simulink model "drone"  (Simulink 6.1)
settings: Solver=ode4  StartTime=0.0  StopTime=15  FixedStep=1e-2  RelTol=1e-3
values from neighbouring files (symbols this model uses):
  Caero = 0    [BACKUP.mat]
  Cfrot = 0.05    [BACKUP.mat]
  Cpert = 0    [BACKUP.mat]
  DZOrientation = 0.05    [BACKUP.mat]
  ExposantFacteurAngulaire = 1    [BACKUP.mat]
  Faero = 0.8    [BACKUP.mat]
  Fpert = 0    [BACKUP.mat]
  FrotorSat = 5    [BACKUP.mat]
  InertieRotor = [0.00025  0  0; 0  0.005  0; 0  0  0.005]    [BACKUP.mat]
  KdAttitude = 0.8    [BACKUP.mat]
  KddAttitude = 0.1    [BACKUP.mat]
  KddPosition = 0.01    [BACKUP.mat]
  KdOrientation = 0.08    [BACKUP.mat]
  KdPosition = 0.5    [BACKUP.mat]
  KiAttitude = 0.001    [BACKUP.mat]
  KiOrientation = 0.02    [BACKUP.mat]
  KiPosition = 0.1    [BACKUP.mat]
  KpAttitude = 20    [BACKUP.mat]
  KpOrientation = 60    [BACKUP.mat]
  KpPosition = 50    [BACKUP.mat]
  l = 0.32    [BACKUP.mat]
  TFrotor = 0.3    [BACKUP.mat]
  Tpert = 1    [BACKUP.mat]
undefined symbols (not defined in the file or in its folder): sigbuilder_block
libraries: mblibv1 x29, simulink x20, aerolibutil x3, aerolibtransform2 x2
settings Model: LastModifiedBy=Vincent
settings OptimizationCC: InlineParams=on
settings DebuggingCC: SolverPrmCheckMsg=warning
settings SimMechanicsCC: VisOnUpdateDiagram=on  VisDuringSimulation=on

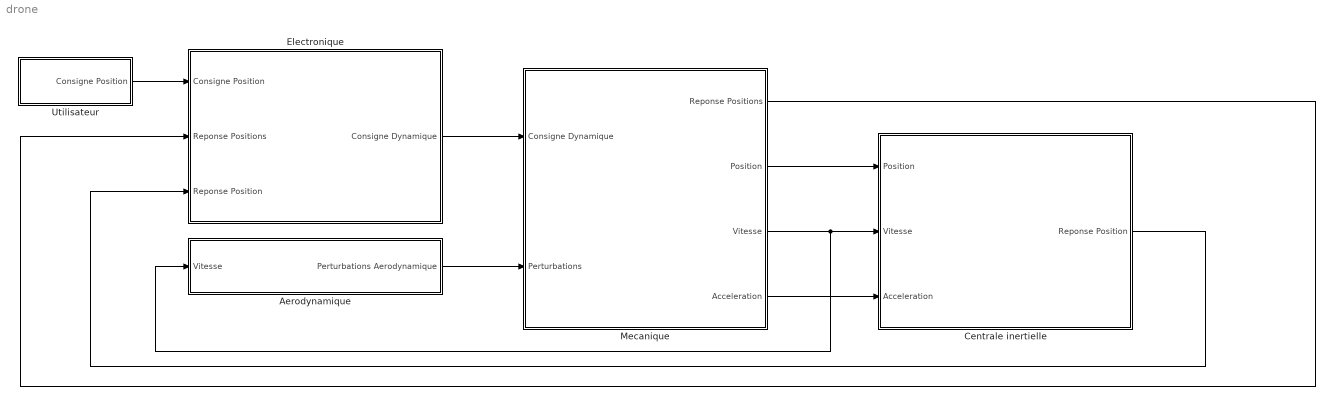
== system drone ==
  Aerodynamique : Subsystem
  Centrale inertielle : Subsystem
  Electronique : Subsystem
  Mecanique : Subsystem
  Utilisateur : Subsystem
  wires:
  Mecanique/1(Reponse Positions) -> Electronique/2(Reponse Positions)
  Electronique/1(Consigne Dynamique) -> Mecanique/1(Consigne Dynamique)
  Aerodynamique/1(Perturbations Aerodynamique) -> Mecanique/2(Perturbations)
  Utilisateur/1(Consigne Position) -> Electronique/1(Consigne Position)
  Mecanique/2(Position) -> Centrale inertielle/1(Position)
  Centrale inertielle/1(Reponse Position) -> Electronique/3(Reponse Position)
  Mecanique/4(Acceleration) -> Centrale inertielle/3(Acceleration)
  Mecanique/3(Vitesse) -> Centrale inertielle/2(Vitesse), Aerodynamique/1(Vitesse)

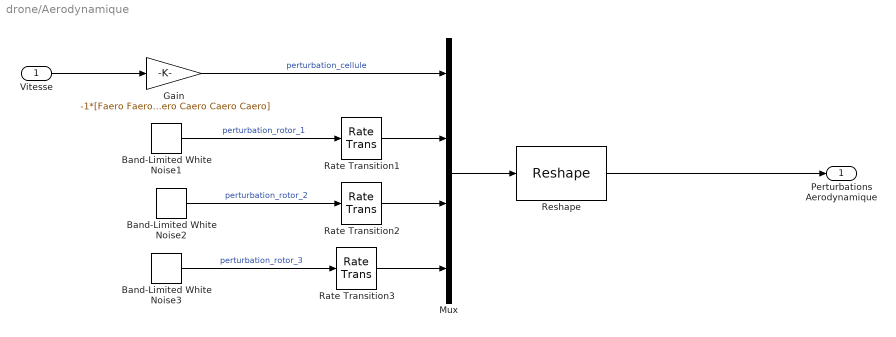
== system drone/Aerodynamique ==
  Vitesse : Inport  Port=1  LatchInput=off
  Band-Limited White Noise1 : simulink/Sources/Band-Limited White Noise  Cov=[Fpert Fpert Fpert Cpert Cpert Cpert]  Ts=Tpert  seed=rand(6,1)*1e5
  Band-Limited White Noise2 : simulink/Sources/Band-Limited White Noise  Cov=[Fpert Fpert Fpert Cpert Cpert Cpert]  Ts=Tpert  seed=rand(6,1)*1e5
  Band-Limited White Noise3 : simulink/Sources/Band-Limited White Noise  Cov=[Fpert Fpert Fpert Cpert Cpert Cpert]  Ts=Tpert  seed=rand(6,1)*1e5
  Gain : Gain  Gain=-1*[Faero Faero Faero Caero Caero Caero]
  Mux : Mux
  Rate Transition1 : RateTransition
  Rate Transition2 : RateTransition
  Rate Transition3 : RateTransition
  Reshape : simulink/Math Operations/Reshape  OutputDimensionality=1-D array  OutputDimensions=[6,4]
  Perturbations Aerodynamique : Outport
      settings: BusObject=perturbations
  wires:
  Band-Limited White Noise1/1 -> Rate Transition1/1  "perturbation_rotor_1"
  Band-Limited White Noise2/1 -> Rate Transition2/1  "perturbation_rotor_2"
  Band-Limited White Noise3/1 -> Rate Transition3/1  "perturbation_rotor_3"
  Gain/1 -> Mux/1  "perturbation_cellule"
  Mux/1 -> Reshape/1
  Reshape/1 -> Perturbations Aerodynamique/1
  Vitesse/1 -> Gain/1
  Rate Transition1/1 -> Mux/2
  Rate Transition2/1 -> Mux/3
  Rate Transition3/1 -> Mux/4

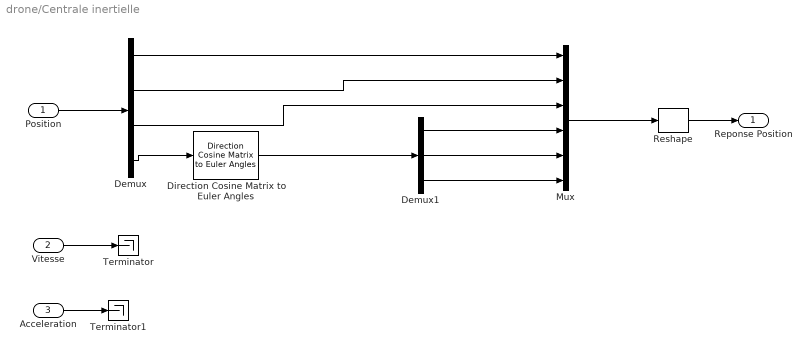
== system drone/Centrale inertielle ==
  Position : Inport  Port=1  LatchInput=off
      settings: BusObject=couples_moteurs
  Vitesse : Inport  Port=2  LatchInput=off
      settings: BusObject=couples_moteurs
  Acceleration : Inport  Port=3  LatchInput=off
      settings: BusObject=couples_moteurs
  Demux : Demux
  Demux1 : Demux  Outputs=3
  Direction Cosine Matrix to Euler Angles : aerolibtransform2/Direction Cosine Matrix to Euler Angles
  Mux : Mux  Inputs=6
  Reshape : simulink/Math Operations/Reshape  OutputDimensionality=1-D array  OutputDimensions=[1,1]
  Terminator : Terminator
  Terminator1 : Terminator
  Reponse Position : Outport
      settings: BusObject=reponse_generale
  wires:
  Position/1 -> Demux/1
  Mux/1 -> Reshape/1
  Reshape/1 -> Reponse Position/1
  Demux/4 -> Direction Cosine Matrix to Euler Angles/1
  Demux/1 -> Mux/1
  Demux/2 -> Mux/2
  Demux/3 -> Mux/3
  Demux1/1 -> Mux/4
  Demux1/2 -> Mux/5
  Demux1/3 -> Mux/6
  Direction Cosine Matrix to Euler Angles/1 -> Demux1/1
  Vitesse/1 -> Terminator/1
  Acceleration/1 -> Terminator1/1

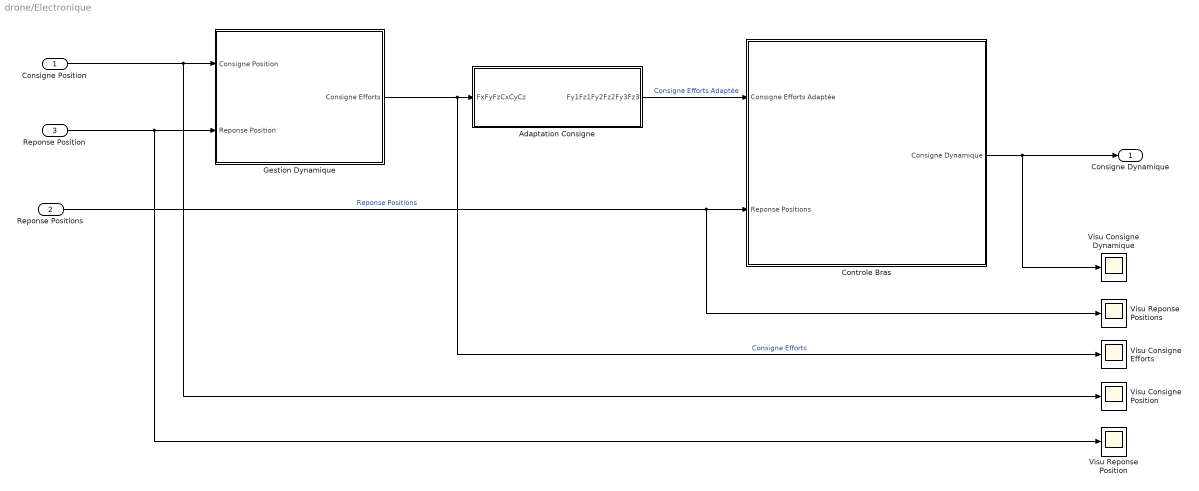
== system drone/Electronique ==
  Consigne Position : Inport  Port=1  LatchInput=off
      settings: BusObject=consigne_generale
  Reponse Positions : Inport  Port=2  LatchInput=off
      settings: BusObject=angles_moteurs
  Reponse Position : Inport  Port=3  LatchInput=off
      settings: BusObject=reponse_generale
  Adaptation Consigne : Subsystem
  Controle Bras : Subsystem
  Gestion Dynamique : Subsystem
  Visu Consigne Dynamique : Scope
      settings: YMin=-6  YMax=6  SaveName=ScopeData3
  Visu Consigne Efforts : Scope
      settings: YMin=-3.5  YMax=4.5  SaveName=ScopeData4
  Visu Consigne Position : Scope
      settings: YMin=-1  YMax=2
  Visu Reponse Position : Scope
      settings: YMin=-1.5  YMax=10
  Visu Reponse Positions : Scope
      settings: YMin=-2  YMax=3.25  SaveName=ScopeData2
  Consigne Dynamique : Outport
      settings: BusObject=couples_moteurs
  wires:
  Consigne Position/1 -> Gestion Dynamique/1(Consigne Position), Visu Consigne Position/1
  Reponse Positions/1 -> Controle Bras/2(Reponse Positions), Visu Reponse Positions/1  "Reponse Positions"
  Adaptation Consigne/1(Fy1Fz1Fy2Fz2Fy3Fz3) -> Controle Bras/1(Consigne Efforts Adaptée)  "Consigne Efforts Adaptée"
  Controle Bras/1(Consigne Dynamique) -> Consigne Dynamique/1, Visu Consigne Dynamique/1
  Gestion Dynamique/1(Consigne Efforts) -> Adaptation Consigne/1(FxFyFzCxCyCz), Visu Consigne Efforts/1  "Consigne Efforts"
  Reponse Position/1 -> Gestion Dynamique/2(Reponse Position), Visu Reponse Position/1

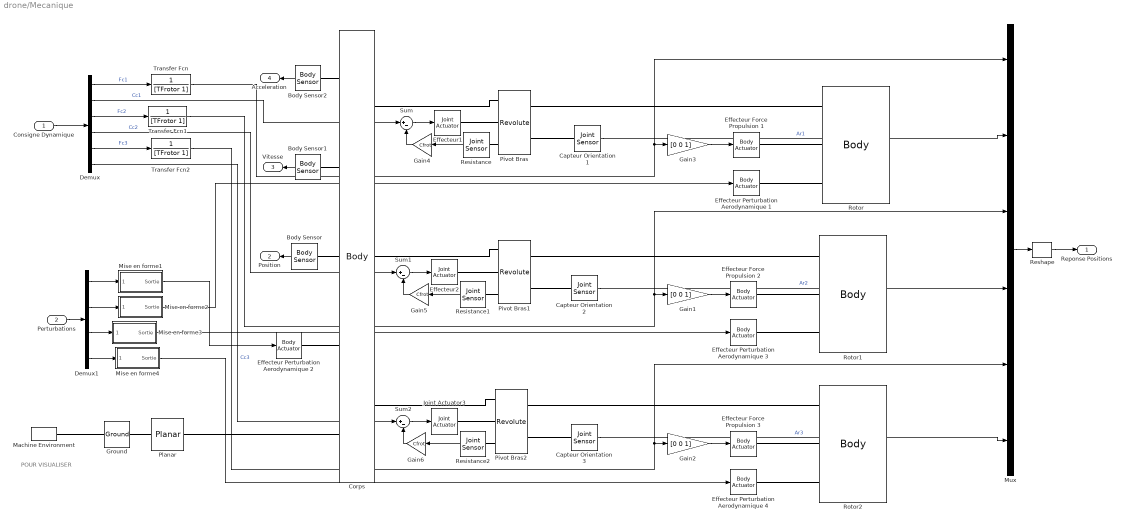
== system drone/Mecanique ==
  note: POUR VISUALISER
  Consigne Dynamique : Inport  Port=1  LatchInput=off
      settings: BusObject=couples_moteurs
  Perturbations : Inport  Port=2  LatchInput=off
      settings: BusObject=perturbations
  Body Sensor : mblibv1/Sensors &  Actuators/Body Sensor  Orientation=left  Opaque=on  PhysicalDomain=Mechanical  PortType=blob  Muxed=on  Pose=on  Angle=on  AngleUnits=deg  ArcVelocity=off  ArcVelocityUnits=deg/s  ArcAcceleration=off  ArcAccelerationUnits=deg/s^2  CoordPosition=on  CoordPositionUnits=m  Velocity=off  VelocityUnits=m/s  Acceleration=off  AccelerationUnits=m/s^2  Quaternion=on  QuaternionDT=off  QuaternionDDT=off  QuaternionUnits=off  OutputVector=[ 3 9 ]  ActiveIO=on  Width=12  DialogClass=MechanicalSensorBlock  ReferenceFrame=Absolute (World)
  Body Sensor1 : mblibv1/Sensors &  Actuators/Body Sensor  Orientation=left  Opaque=on  PhysicalDomain=Mechanical  PortType=blob  Muxed=on  Pose=off  Angle=on  AngleUnits=deg  ArcVelocity=on  ArcVelocityUnits=rad/s  ArcAcceleration=off  ArcAccelerationUnits=deg/s^2  CoordPosition=off  CoordPositionUnits=m  Velocity=on  VelocityUnits=m/s  Acceleration=off  AccelerationUnits=m/s^2  Quaternion=on  QuaternionDT=off  QuaternionDDT=off  QuaternionUnits=off  OutputVector=[ 3 3 ]  ActiveIO=on  Width=6  DialogClass=MechanicalSensorBlock  ReferenceFrame=Absolute (World)
  Body Sensor2 : mblibv1/Sensors &  Actuators/Body Sensor  Orientation=left  Opaque=on  PhysicalDomain=Mechanical  PortType=blob  Muxed=on  Pose=off  Angle=on  AngleUnits=deg  ArcVelocity=off  ArcVelocityUnits=deg/s  ArcAcceleration=on  ArcAccelerationUnits=rad/s^2  CoordPosition=off  CoordPositionUnits=m  Velocity=off  VelocityUnits=m/s  Acceleration=on  AccelerationUnits=m/s^2  Quaternion=on  QuaternionDT=off  QuaternionDDT=off  QuaternionUnits=off  OutputVector=[ 3 3 ]  ActiveIO=on  Width=6  DialogClass=MechanicalSensorBlock  ReferenceFrame=Absolute (World)
  Capteur Orientation 1 : mblibv1/Sensors &  Actuators/Joint Sensor  Opaque=on  PhysicalDomain=Mechanical  PortType=blob  Muxed=on  Pose=off  Angle=on  AngleUnits=rad  ArcVelocity=off  ArcVelocityUnits=rad/s  ArcAcceleration=off  ArcAccelerationUnits=rad/s^2  CoordPosition=on  CoordPositionUnits=m  Velocity=off  VelocityUnits=m/s  Acceleration=off  AccelerationUnits=m/s^2  Quaternion=on  QuaternionDT=off  QuaternionDDT=off  QuaternionUnits=off  OutputVector=[ 1 ]  ActiveIO=on  Width=1  DialogClass=MechanicalSensorBlock  Primitive=R1  Force=off  ForceUnits=N  Torque=off  TorqueUnits=N-m  ReferenceFrame=Absolute (INERTIAL)  ReactionSensedSide=Base  ReactionReferenceFrame=Local (Body CS)  ReactionForce=off  ReactionForceUnits=N  ReactionMoment=off  ReactionMomentUnits=N-m
  Capteur Orientation 2 : mblibv1/Sensors &  Actuators/Joint Sensor  Opaque=on  PhysicalDomain=Mechanical  PortType=blob  Muxed=on  Pose=off  Angle=on  AngleUnits=rad  ArcVelocity=off  ArcVelocityUnits=rad/s  ArcAcceleration=off  ArcAccelerationUnits=rad/s^2  CoordPosition=on  CoordPositionUnits=m  Velocity=off  VelocityUnits=m/s  Acceleration=off  AccelerationUnits=m/s^2  Quaternion=on  QuaternionDT=off  QuaternionDDT=off  QuaternionUnits=off  OutputVector=[ 1 ]  ActiveIO=on  Width=1  DialogClass=MechanicalSensorBlock  Primitive=R1  Force=off  ForceUnits=N  Torque=off  TorqueUnits=N-m  ReferenceFrame=Absolute (INERTIAL)  ReactionSensedSide=Base  ReactionReferenceFrame=Local (Body CS)  ReactionForce=off  ReactionForceUnits=N  ReactionMoment=off  ReactionMomentUnits=N-m
  Capteur Orientation 3 : mblibv1/Sensors &  Actuators/Joint Sensor  Opaque=on  PhysicalDomain=Mechanical  PortType=blob  Muxed=on  Pose=off  Angle=on  AngleUnits=rad  ArcVelocity=off  ArcVelocityUnits=rad/s  ArcAcceleration=off  ArcAccelerationUnits=rad/s^2  CoordPosition=on  CoordPositionUnits=m  Velocity=off  VelocityUnits=m/s  Acceleration=off  AccelerationUnits=m/s^2  Quaternion=on  QuaternionDT=off  QuaternionDDT=off  QuaternionUnits=off  OutputVector=[ 1 ]  ActiveIO=on  Width=1  DialogClass=MechanicalSensorBlock  Primitive=R1  Force=off  ForceUnits=N  Torque=off  TorqueUnits=N-m  ReferenceFrame=Absolute (INERTIAL)  ReactionSensedSide=Base  ReactionReferenceFrame=Local (Body CS)  ReactionForce=off  ReactionForceUnits=N  ReactionMoment=off  ReactionMomentUnits=N-m
  Corps : mblibv1/Bodies/Body  PhysicalDomain=mechanical  SubClassName=Unknown  LeftPortType=workingframe  RightPortType=workingframe  LConnTagsString=CS4|CS5|CS6|CS7|CG  RConnTagsString=CS1|CS2|CS3  DialogClass=MechanicalBodyBlock  Mass=0.2  MassUnits=kg  InertiaUnits=kg*m^2  Inertia=eye(3)  Shape=Cylinder  ShapeDims=[1 1]  ShapeUnits=m  ShapeUse=false  Density=1  DensityUnits=kg/m^3  DensityUse=false  CG=Left$CG$[0 0 0]$ADJOINING$ADJOINING$m$[0 0 0]$Euler X-Y-Z$deg$ADJOINING$true  WorkingFrames=Right$CS1$[0 0 0]$CG$CG$m$[0 0 0]$Euler Z-Y-X$deg$CG$true#Right$CS2$[0 0 0]$CG$CG$m$[120 0 0]$Euler Z-Y-X$deg$CG$true#Right$CS3$[0 0 0]$CG$CG$m$[240 0 0]$Euler Z-Y-X$deg$CG$true#Left$CS4$[0 0 0]$CG$CG$m$[0 0 0]$Euler X-Y-Z$deg$WORLD$true#Left$CS5$[0 0 0]$CG$CG$m$[0 0 0]$Euler X-Y-Z$deg$WORLD$true#Left$CS6$[0 0 0]$CG$CG$m$[0 0 0]$Euler X-Y-Z$deg$WORLD$true#Left$CS7$[0 0 0]$CG$CG$m$[0 0 0]$Euler X-Y-Z$deg$WORLD$true
  Demux : Demux  Outputs=6
  Demux1 : Demux
  Effecteur Force Propulsion 1 : mblibv1/Sensors &  Actuators/Body Actuator  Opaque=on  PhysicalDomain=Mechanical  PortType=blob  ActuationStyle=Force  AngleUnits=deg  ArcVelocityUnits=deg/s  ArcAccelerationUnits=deg/s^2  CoordPositionUnits=m  VelocityUnits=m/s  AccelerationUnits=m/s^2  ForceUnits=N  TorqueUnits=N-m  ActiveIO=on  Width=3  DialogClass=MechanicalActuatorBlock  ReferenceFrame=Local (Body CS)  Angle=off  CoordPosition=on  Force=on  Torque=off
  Effecteur Force Propulsion 2 : mblibv1/Sensors &  Actuators/Body Actuator  Opaque=on  PhysicalDomain=Mechanical  PortType=blob  ActuationStyle=Force  AngleUnits=deg  ArcVelocityUnits=deg/s  ArcAccelerationUnits=deg/s^2  CoordPositionUnits=m  VelocityUnits=m/s  AccelerationUnits=m/s^2  ForceUnits=N  TorqueUnits=N-m  ActiveIO=on  Width=3  DialogClass=MechanicalActuatorBlock  ReferenceFrame=Local (Body CS)  Angle=off  CoordPosition=on  Force=on  Torque=off
  Effecteur Force Propulsion 3 : mblibv1/Sensors &  Actuators/Body Actuator  Opaque=on  PhysicalDomain=Mechanical  PortType=blob  ActuationStyle=Force  AngleUnits=deg  ArcVelocityUnits=deg/s  ArcAccelerationUnits=deg/s^2  CoordPositionUnits=m  VelocityUnits=m/s  AccelerationUnits=m/s^2  ForceUnits=N  TorqueUnits=N-m  ActiveIO=on  Width=3  DialogClass=MechanicalActuatorBlock  ReferenceFrame=Local (Body CS)  Angle=off  CoordPosition=on  Force=on  Torque=off
  Effecteur Perturbation Aerodynamique 1 : mblibv1/Sensors &  Actuators/Body Actuator  Opaque=on  PhysicalDomain=Mechanical  PortType=blob  ActuationStyle=Force  AngleUnits=deg  ArcVelocityUnits=deg/s  ArcAccelerationUnits=deg/s^2  CoordPositionUnits=m  VelocityUnits=m/s  AccelerationUnits=m/s^2  ForceUnits=N  TorqueUnits=N-m  ActiveIO=on  Width=6  DialogClass=MechanicalActuatorBlock  ReferenceFrame=Local (Body CS)  Angle=off  CoordPosition=on  Force=on  Torque=on
  Effecteur Perturbation Aerodynamique 2 : mblibv1/Sensors &  Actuators/Body Actuator  Opaque=on  PhysicalDomain=Mechanical  PortType=blob  ActuationStyle=Force  AngleUnits=deg  ArcVelocityUnits=deg/s  ArcAccelerationUnits=deg/s^2  CoordPositionUnits=m  VelocityUnits=m/s  AccelerationUnits=m/s^2  ForceUnits=N  TorqueUnits=N-m  ActiveIO=on  Width=6  DialogClass=MechanicalActuatorBlock  ReferenceFrame=Absolute (World)  Angle=off  CoordPosition=on  Force=on  Torque=on
  Effecteur Perturbation Aerodynamique 3 : mblibv1/Sensors &  Actuators/Body Actuator  Opaque=on  PhysicalDomain=Mechanical  PortType=blob  ActuationStyle=Force  AngleUnits=deg  ArcVelocityUnits=deg/s  ArcAccelerationUnits=deg/s^2  CoordPositionUnits=m  VelocityUnits=m/s  AccelerationUnits=m/s^2  ForceUnits=N  TorqueUnits=N-m  ActiveIO=on  Width=6  DialogClass=MechanicalActuatorBlock  ReferenceFrame=Local (Body CS)  Angle=off  CoordPosition=on  Force=on  Torque=on
  Effecteur Perturbation Aerodynamique 4 : mblibv1/Sensors &  Actuators/Body Actuator  Opaque=on  PhysicalDomain=Mechanical  PortType=blob  ActuationStyle=Force  AngleUnits=deg  ArcVelocityUnits=deg/s  ArcAccelerationUnits=deg/s^2  CoordPositionUnits=m  VelocityUnits=m/s  AccelerationUnits=m/s^2  ForceUnits=N  TorqueUnits=N-m  ActiveIO=on  Width=6  DialogClass=MechanicalActuatorBlock  ReferenceFrame=Local (Body CS)  Angle=off  CoordPosition=on  Force=on  Torque=on
  Effecteur1 : mblibv1/Sensors &  Actuators/Joint Actuator  Opaque=on  PhysicalDomain=Mechanical  PortType=blob  ActuationStyle=Force  AngleUnits=deg  ArcVelocityUnits=deg/s  ArcAccelerationUnits=deg/s^2  CoordPositionUnits=m  VelocityUnits=m/s  AccelerationUnits=m/s^2  ForceUnits=N  TorqueUnits=N-m  ActiveIO=on  Width=1  DialogClass=MechanicalActuatorBlock  Primitive=R1  ReferenceFrame=Absolute (INERTIAL)
  Effecteur2 : mblibv1/Sensors &  Actuators/Joint Actuator  Opaque=on  PhysicalDomain=Mechanical  PortType=blob  ActuationStyle=Force  AngleUnits=deg  ArcVelocityUnits=deg/s  ArcAccelerationUnits=deg/s^2  CoordPositionUnits=m  VelocityUnits=m/s  AccelerationUnits=m/s^2  ForceUnits=N  TorqueUnits=N-m  ActiveIO=on  Width=1  DialogClass=MechanicalActuatorBlock  Primitive=R1  ReferenceFrame=Absolute (INERTIAL)
  Gain1 : Gain  Gain=[0 0 1]
  Gain2 : Gain  Gain=[0 0 1]
  Gain3 : Gain  Gain=[0 0 1]
  Gain4 : Gain  Orientation=left  Gain=Cfrot
  Gain5 : Gain  Orientation=left  Gain=Cfrot
  Gain6 : Gain  Orientation=left  Gain=Cfrot
  Ground : mblibv1/Bodies/Ground  Opaque=on  LeftPortType=env  RightPortType=workingframe  PhysicalDomain=Mechanical  DialogClass=GroundBlock  CoordPosition=[0 0 0]  CoordPositionUnits=m  StateVectorMgrId=-1  MachineId=[1 0]  ShowEnvPort=on
  Joint Actuator3 : mblibv1/Sensors &  Actuators/Joint Actuator  Opaque=on  PhysicalDomain=Mechanical  PortType=blob  ActuationStyle=Force  AngleUnits=deg  ArcVelocityUnits=deg/s  ArcAccelerationUnits=deg/s^2  CoordPositionUnits=m  VelocityUnits=m/s  AccelerationUnits=m/s^2  ForceUnits=N  TorqueUnits=N-m  ActiveIO=on  Width=1  DialogClass=MechanicalActuatorBlock  Primitive=R1  ReferenceFrame=Absolute (INERTIAL)
  Machine Environment : mblibv1/Bodies/Machine Environment  Tag=Factory ground  DialogController=MECH.DialogSource  Opaque=on  PortType=env  PhysicalDomain=Mechanical  DialogTemplateClass=MECH.MachineEnvironment  SyncWhenCopied=off  Gravity=[0 0 -9.81]  GravityUnits=m/s^2  GravityAsSignal=off  Dimensionality=3D Only  AnalysisType=Forward dynamics  LinearAssemblyTolerance=1e-3  LinearAssemblyToleranceUnits=m  AngularAssemblyTolerance=1e-3  AngularAssemblyToleranceUnits=rad  ConstraintSolverType=Stabilizing  ConstraintRelTolerance=1e-4  ConstraintAbsTolerance=1e-4  UseRobustSingularityHandling=off  StatePerturbationType=Fixed  PerturbationSize=1e-5  VisualizeMachine=on
  Mise en forme1 : Subsystem
  Mise en forme2 : Subsystem
  Mise en forme3 : Subsystem
  Mise en forme4 : Subsystem
  Mux : Mux  Inputs=6
  Pivot Bras : mblibv1/Joints/Revolute  PhysicalDomain=mechanical  SubClassName=Unknown  LeftPortType=blob  RightPortType=blob  LConnTagsString=__newl0|SA1|SA2  RConnTagsString=__newr0|SA1  NumSAPorts=3  CutJoint=off  MarkAsCut=off  Primitives=revolute  PrimitiveProps=R1$Base$[1 0 0]$revolute  DialogClass=JointBlock
  Pivot Bras1 : mblibv1/Joints/Revolute  PhysicalDomain=mechanical  SubClassName=Unknown  LeftPortType=blob  RightPortType=blob  LConnTagsString=__newl0|SA1|SA2  RConnTagsString=__newr0|SA1  NumSAPorts=3  CutJoint=off  MarkAsCut=off  Primitives=revolute  PrimitiveProps=R1$Base$[1 0 0]$revolute  DialogClass=JointBlock
  Pivot Bras2 : mblibv1/Joints/Revolute  PhysicalDomain=mechanical  SubClassName=Unknown  LeftPortType=blob  RightPortType=blob  LConnTagsString=__newl0|SA1|SA2  RConnTagsString=__newr0|SA1  NumSAPorts=3  CutJoint=off  MarkAsCut=off  Primitives=revolute  PrimitiveProps=R1$Base$[1 0 0]$revolute  DialogClass=JointBlock
  Planar : mblibv1/Joints/Planar  PhysicalDomain=mechanical  SubClassName=Unknown  LeftPortType=blob  RightPortType=blob  LConnTagsString=__newl0  RConnTagsString=__newr0  NumSAPorts=0  CutJoint=off  MarkAsCut=off  Primitives=prismatic_prismatic_revolute  PrimitiveProps=P1$INERTIAL$[1 0 0]$prismatic#P2$INERTIAL$[0 1 0]$prismatic#R1$INERTIAL$[0 0 1]$revolute  DialogClass=JointBlock
  Reshape : simulink/Math Operations/Reshape  OutputDimensionality=1-D array  OutputDimensions=[1,1]
  Resistance : mblibv1/Sensors &  Actuators/Joint Sensor  Orientation=left  Opaque=on  PhysicalDomain=Mechanical  PortType=blob  Muxed=on  Pose=off  Angle=off  AngleUnits=rad  ArcVelocity=on  ArcVelocityUnits=rad/s  ArcAcceleration=off  ArcAccelerationUnits=rad/s^2  CoordPosition=on  CoordPositionUnits=m  Velocity=off  VelocityUnits=m/s  Acceleration=off  AccelerationUnits=m/s^2  Quaternion=on  QuaternionDT=off  QuaternionDDT=off  QuaternionUnits=off  OutputVector=[ 1 ]  ActiveIO=on  Width=1  DialogClass=MechanicalSensorBlock  Primitive=R1  Force=off  ForceUnits=N  Torque=off  TorqueUnits=N-m  ReferenceFrame=Absolute (INERTIAL)  ReactionSensedSide=Base  ReactionReferenceFrame=Local (Body CS)  ReactionForce=off  ReactionForceUnits=N  ReactionMoment=off  ReactionMomentUnits=N-m
  Resistance1 : mblibv1/Sensors &  Actuators/Joint Sensor  Orientation=left  Opaque=on  PhysicalDomain=Mechanical  PortType=blob  Muxed=on  Pose=off  Angle=off  AngleUnits=rad  ArcVelocity=on  ArcVelocityUnits=rad/s  ArcAcceleration=off  ArcAccelerationUnits=rad/s^2  CoordPosition=on  CoordPositionUnits=m  Velocity=off  VelocityUnits=m/s  Acceleration=off  AccelerationUnits=m/s^2  Quaternion=on  QuaternionDT=off  QuaternionDDT=off  QuaternionUnits=off  OutputVector=[ 1 ]  ActiveIO=on  Width=1  DialogClass=MechanicalSensorBlock  Primitive=R1  Force=off  ForceUnits=N  Torque=off  TorqueUnits=N-m  ReferenceFrame=Absolute (INERTIAL)  ReactionSensedSide=Base  ReactionReferenceFrame=Local (Body CS)  ReactionForce=off  ReactionForceUnits=N  ReactionMoment=off  ReactionMomentUnits=N-m
  Resistance2 : mblibv1/Sensors &  Actuators/Joint Sensor  Orientation=left  Opaque=on  PhysicalDomain=Mechanical  PortType=blob  Muxed=on  Pose=off  Angle=off  AngleUnits=rad  ArcVelocity=on  ArcVelocityUnits=rad/s  ArcAcceleration=off  ArcAccelerationUnits=rad/s^2  CoordPosition=on  CoordPositionUnits=m  Velocity=off  VelocityUnits=m/s  Acceleration=off  AccelerationUnits=m/s^2  Quaternion=on  QuaternionDT=off  QuaternionDDT=off  QuaternionUnits=off  OutputVector=[ 1 ]  ActiveIO=on  Width=1  DialogClass=MechanicalSensorBlock  Primitive=R1  Force=off  ForceUnits=N  Torque=off  TorqueUnits=N-m  ReferenceFrame=Absolute (INERTIAL)  ReactionSensedSide=Base  ReactionReferenceFrame=Local (Body CS)  ReactionForce=off  ReactionForceUnits=N  ReactionMoment=off  ReactionMomentUnits=N-m
  Rotor : mblibv1/Bodies/Body  PhysicalDomain=mechanical  SubClassName=Unknown  LeftPortType=workingframe  RightPortType=workingframe  LConnTagsString=CS1|CS2|CS3  DialogClass=MechanicalBodyBlock  Mass=0.1  MassUnits=kg  InertiaUnits=kg*m^2  Inertia=InertieRotor  Shape=Cylinder  ShapeDims=[1 1]  ShapeUnits=m  ShapeUse=false  Density=1  DensityUnits=kg/m^3  DensityUse=false  CG=Left$CG$l*[1 0 0]$CS1$CS1$m$[0 0 0]$Euler X-Y-Z$deg$CS1$false  WorkingFrames=Left$CS1$[0 0 0]$ADJOINING$ADJOINING$m$[0 0 0]$Euler X-Y-Z$deg$ADJOINING$true#Left$CS2$l*[1 0 0]$CS1$CS1$m$[0 0 0]$Euler X-Y-Z$deg$CS1$true#Left$CS3$l*[1 0 0]$CS1$CS1$m$[0 0 0]$Euler X-Y-Z$deg$CS1$true
  Rotor1 : mblibv1/Bodies/Body  PhysicalDomain=mechanical  SubClassName=Unknown  LeftPortType=workingframe  RightPortType=workingframe  LConnTagsString=CS1|CS2|CS3  DialogClass=MechanicalBodyBlock  Mass=0.1  MassUnits=kg  InertiaUnits=kg*m^2  Inertia=InertieRotor  Shape=Cylinder  ShapeDims=[1 1]  ShapeUnits=m  ShapeUse=false  Density=1  DensityUnits=kg/m^3  DensityUse=false  CG=Left$CG$l*[1 0 0]$CS1$CS1$m$[0 0 0]$Euler X-Y-Z$deg$CS1$false  WorkingFrames=Left$CS1$[0 0 0]$ADJOINING$ADJOINING$m$[0 0 0]$Euler X-Y-Z$deg$ADJOINING$true#Left$CS2$l*[1 0 0]$CS1$CS1$m$[0 0 0]$Euler X-Y-Z$deg$CS1$true#Left$CS3$l*[1 0 0]$CS1$CS1$m$[0 0 0]$Euler X-Y-Z$deg$CS1$true
  Rotor2 : mblibv1/Bodies/Body  PhysicalDomain=mechanical  SubClassName=Unknown  LeftPortType=workingframe  RightPortType=workingframe  LConnTagsString=CS1|CS2|CS3  DialogClass=MechanicalBodyBlock  Mass=0.1  MassUnits=kg  InertiaUnits=kg*m^2  Inertia=InertieRotor  Shape=Cylinder  ShapeDims=[1 1]  ShapeUnits=m  ShapeUse=false  Density=1  DensityUnits=kg/m^3  DensityUse=false  CG=Left$CG$l*[1 0 0]$CS1$CS1$m$[0 0 0]$Euler X-Y-Z$deg$CS1$false  WorkingFrames=Left$CS1$[0 0 0]$ADJOINING$ADJOINING$m$[0 0 0]$Euler X-Y-Z$deg$ADJOINING$true#Left$CS2$l*[1 0 0]$CS1$CS1$m$[0 0 0]$Euler X-Y-Z$deg$CS1$true#Left$CS3$l*[1 0 0]$CS1$CS1$m$[0 0 0]$Euler X-Y-Z$deg$CS1$true
  Sum : Sum  Inputs=|+-
  Sum1 : Sum  Inputs=|+-
  Sum2 : Sum  Inputs=|+-
  Transfer Fcn : TransferFcn  Denominator=[TFrotor 1]
  Transfer Fcn1 : TransferFcn  Denominator=[TFrotor 1]
  Transfer Fcn2 : TransferFcn  Denominator=[TFrotor 1]
  Reponse Positions : Outport
      settings: BusObject=angles_moteurs
  Position : Outport  Orientation=left  Port=2
      settings: BusObject=angles_moteurs
  Vitesse : Outport  Orientation=left  Port=3
      settings: BusObject=angles_moteurs
  Acceleration : Outport  Orientation=left  Port=4
      settings: BusObject=angles_moteurs
  wires:
  Consigne Dynamique/1 -> Demux/1
  Demux/2 -> Sum/1  "Cc1"
  Demux/1 -> Transfer Fcn/1  "Fc1"
  Demux/4 -> Sum1/1  "Cc2"
  Demux/3 -> Transfer Fcn1/1  "Fc2"
  Demux/5 -> Transfer Fcn2/1  "Fc3"
  Demux/6 -> Sum2/1  "Cc3"
  Reshape/1 -> Reponse Positions/1
  Capteur Orientation 3/1 -> Mux/6  "Ar3"
  Capteur Orientation 2/1 -> Mux/4  "Ar2"
  Capteur Orientation 1/1 -> Mux/2  "Ar1"
  Mux/1 -> Reshape/1
  Gain2/1 -> Effecteur Force Propulsion 3/1
  Gain1/1 -> Effecteur Force Propulsion 2/1
  Gain3/1 -> Effecteur Force Propulsion 1/1
  Perturbations/1 -> Demux1/1
  Demux1/2 -> Mise en forme2/1(Entree)
  Demux1/3 -> Mise en forme3/1(Entree)
  Demux1/4 -> Mise en forme4/1(Entree)
  Demux1/1 -> Mise en forme1/1(Entree)
  Sum/1 -> Effecteur1/1
  Resistance/1 -> Gain4/1
  Gain4/1 -> Sum/2
  Gain5/1 -> Sum1/2
  Resistance1/1 -> Gain5/1
  Sum1/1 -> Effecteur2/1
  Gain6/1 -> Sum2/2
  Resistance2/1 -> Gain6/1
  Sum2/1 -> Joint Actuator3/1
  Transfer Fcn/1 -> Mux/1, Gain3/1
  Transfer Fcn1/1 -> Mux/3, Gain1/1
  Transfer Fcn2/1 -> Mux/5, Gain2/1
  Body Sensor/1 -> Position/1
  Body Sensor1/1 -> Vitesse/1
  Body Sensor2/1 -> Acceleration/1
  Mise en forme1/1(Sortie) -> Effecteur Perturbation Aerodynamique 2/1
  Mise en forme2/1(Sortie) -> Effecteur Perturbation Aerodynamique 1/1
  Mise en forme3/1(Sortie) -> Effecteur Perturbation Aerodynamique 3/1
  Mise en forme4/1(Sortie) -> Effecteur Perturbation Aerodynamique 4/1
  connections:
  Corps/RConn1 -- Pivot Bras/LConn1
  Pivot Bras/RConn1 -- Rotor/LConn1
  Effecteur Force Propulsion 1/RConn1 -- Rotor/LConn2
  Effecteur Perturbation Aerodynamique 1/RConn1 -- Rotor/LConn3
  Pivot Bras/RConn2 -- Capteur Orientation 1/LConn1
  Ground/RConn1 -- Planar/LConn1
  Planar/RConn1 -- Corps/LConn5
  Machine Environment/RConn1 -- Ground/LConn1
  Effecteur1/RConn1 -- Pivot Bras/LConn2
  Pivot Bras1/RConn1 -- Rotor1/LConn1
  Effecteur Force Propulsion 2/RConn1 -- Rotor1/LConn2
  Effecteur Perturbation Aerodynamique 3/RConn1 -- Rotor1/LConn3
  Pivot Bras1/RConn2 -- Capteur Orientation 2/LConn1
  Effecteur2/RConn1 -- Pivot Bras1/LConn2
  Pivot Bras2/RConn1 -- Rotor2/LConn1
  Effecteur Force Propulsion 3/RConn1 -- Rotor2/LConn2
  Effecteur Perturbation Aerodynamique 4/RConn1 -- Rotor2/LConn3
  Pivot Bras2/RConn2 -- Capteur Orientation 3/LConn1
  Joint Actuator3/RConn1 -- Pivot Bras2/LConn2
  Corps/RConn2 -- Pivot Bras1/LConn1
  Corps/RConn3 -- Pivot Bras2/LConn1
  Pivot Bras/LConn3 -- Resistance/LConn1
  Pivot Bras1/LConn3 -- Resistance1/LConn1
  Pivot Bras2/LConn3 -- Resistance2/LConn1
  Effecteur Perturbation Aerodynamique 2/RConn1 -- Corps/LConn4
  Corps/LConn3 -- Body Sensor/LConn1
  Body Sensor1/LConn1 -- Corps/LConn2
  Body Sensor2/LConn1 -- Corps/LConn1

== system drone/Utilisateur ==
  Generateur F : Subsystem  Tag=STV Subsys  LoadFcn=sigbuilder_block('load',[0 42 1080 574.5 ]);  StartFcn=sigbuilder_block('start');  StopFcn=sigbuilder_block('stop');  ClipboardFcn=sigbuilder_block('clipboard');  mask(Sigbuilder block){}
      mask help: Sigbuilder GUI
      mask init:
      | if ~strcmp(get_param(bdroot(gcbh),'SimulationStatus'),'stopped') tuvar = sigbuilder_block('maskInit'); end
      settings: CopyFcn=sigbuilder_block('copy');  DeleteFcn=sigbuilder_block('delete');  ModelCloseFcn=sigbuilder_block('modelClose');  PreSaveFcn=sigbuilder_block('preSave');  NameChangeFcn=sigbuilder_block('namechange');  OpenFcn=sigbuilder_block('open',[0 42 1080 574.5 ]);  CloseFcn=sigbuilder_block('close');
      mask Display: plot(0,0,100,100,[10,10,40,40,10],[80,20,20,80,80],[40,10],[50,50], [40,27,10],[65,72,56],[40,25,25,10],[28,28,43,43]);
  Mux : Mux  Inputs=6
  Reshape2 : simulink/Math Operations/Reshape  OutputDimensionality=1-D array  OutputDimensions=[1,1]
  Consigne Position : Outport
      settings: BusObject=consigne_generale
  wires:
  Mux/1 -> Reshape2/1
  Reshape2/1 -> Consigne Position/1
  Generateur F/1(X) -> Mux/1
  Generateur F/2(Y) -> Mux/2
  Generateur F/3(Z) -> Mux/3
  Generateur F/4(Phi) -> Mux/4
  Generateur F/5(Theta) -> Mux/5
  Generateur F/6(Psi) -> Mux/6

== system drone/Electronique/Adaptation Consigne ==
  FxFyFzCxCyCz : Inport  Port=1  LatchInput=off
  Matrice Correction : Constant  Value=[-1 -1 1 1/l 1/l 1/l]
  Matrice Transformation : Constant  Value=(1/3)*[0 2 0 0 0 1; 0 0 1 0 2 0; -sqrt(3) -1 0 0 0 1; 0 0 1 -sqrt(3) -1 0; sqrt(3) -1 0 0 0 1; 0 0 1 sqrt(3) -1 0]  VectorParams1D=off
  Product : Product  Multiplication=Matrix(*)  RndMeth=Zero
  Product1 : Product  RndMeth=Zero
  Fy1Fz1Fy2Fz2Fy3Fz3 : Outport
  wires:
  Product/1 -> Fy1Fz1Fy2Fz2Fy3Fz3/1
  Matrice Transformation/1 -> Product/1
  Matrice Correction/1 -> Product1/2
  FxFyFzCxCyCz/1 -> Product1/1
  Product1/1 -> Product/2

== system drone/Electronique/Controle Bras ==
  Consigne Efforts Adaptée : Inport  Port=1  LatchInput=off
  Reponse Positions : Inport  Port=2  LatchInput=off
  Controle Bras1 : Subsystem
  Controle Bras2 : Subsystem
  Controle Bras3 : Subsystem
  Demux1 : Demux  Outputs=6
  Demux2 : Demux  Outputs=6
  Mux : Mux  Inputs=6
  Reshape : simulink/Math Operations/Reshape  OutputDimensionality=1-D array  OutputDimensions=[1,1]
  Consigne Dynamique : Outport
  wires:
  Demux1/1 -> Controle Bras1/3(Fr)  "Fr1"
  Demux1/2 -> Controle Bras1/4(Ar)  "Ar1"
  Demux1/3 -> Controle Bras2/3(Fr)  "Fr2"
  Demux1/4 -> Controle Bras2/4(Ar)  "Ar2"
  Demux1/5 -> Controle Bras3/3(Fr)  "Fr3"
  Demux1/6 -> Controle Bras3/4(Ar)  "Ar3"
  Demux2/3 -> Controle Bras2/1(Fyc)  "Fyc2"
  Demux2/4 -> Controle Bras2/2(Fzc)  "Fzc2"
  Demux2/5 -> Controle Bras3/1(Fyc)  "Fyc3"
  Demux2/6 -> Controle Bras3/2(Fzc)  "Fzc3"
  Demux2/1 -> Controle Bras1/1(Fyc)  "Fyc1"
  Demux2/2 -> Controle Bras1/2(Fzc)  "Fzc1"
  Reponse Positions/1 -> Demux1/1
  Consigne Efforts Adaptée/1 -> Demux2/1
  Controle Bras1/1(Fc) -> Mux/1  "Fc1"
  Controle Bras1/2(Cc) -> Mux/2  "Cc1"
  Controle Bras2/1(Fc) -> Mux/3  "Fc2"
  Controle Bras2/2(Cc) -> Mux/4  "Cc2"
  Controle Bras3/1(Fc) -> Mux/5  "Fc3"
  Controle Bras3/2(Cc) -> Mux/6  "Cc3"
  Mux/1 -> Reshape/1
  Reshape/1 -> Consigne Dynamique/1

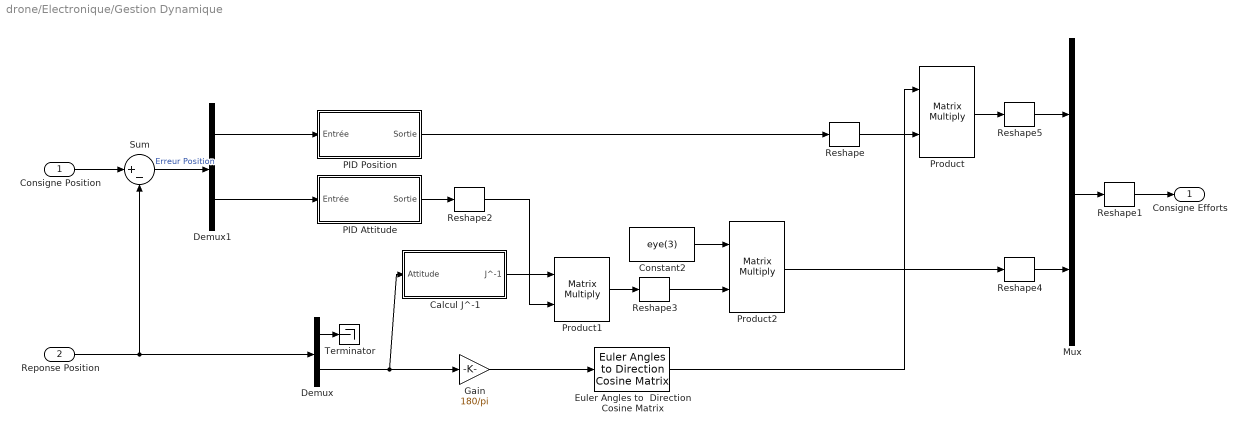
== system drone/Electronique/Gestion Dynamique ==
  Consigne Position : Inport  Port=1  LatchInput=off
  Reponse Position : Inport  Port=2  LatchInput=off
  Calcul J^-1 : Subsystem
  Constant2 : Constant  Value=eye(3)  VectorParams1D=off
  Demux : Demux  Outputs=2
  Demux1 : Demux  Outputs=2
  Euler Angles to  Direction Cosine Matrix : aerolibtransform2/Euler Angles to  Direction Cosine Matrix
  Gain : Gain  Gain=180/pi
  Mux : Mux  Inputs=2
  PID Attitude : Subsystem
  PID Position : Subsystem
  Product : Product  Multiplication=Matrix(*)  RndMeth=Zero
  Product1 : Product  Multiplication=Matrix(*)  RndMeth=Zero
  Product2 : Product  Multiplication=Matrix(*)  RndMeth=Zero
  Reshape{,1..5} (6 alike) : simulink/Math Operations/Reshape  OutputDimensionality=1-D array  OutputDimensions=[1,1]
  Sum : Sum  Inputs=|+-
  Terminator : Terminator
  Consigne Efforts : Outport
  wires:
  Consigne Position/1 -> Sum/1
  Reponse Position/1 -> Sum/2, Demux/1
  Sum/1 -> Demux1/1  "Erreur Position"
  Demux/2 -> Gain/1, Calcul J^-1/1(Attitude)
  Demux/1 -> Terminator/1
  Demux1/1 -> PID Position/1(Entrée)
  Mux/1 -> Reshape1/1
  Reshape1/1 -> Consigne Efforts/1
  Product/1 -> Reshape5/1
  Reshape2/1 -> Product1/2
  Demux1/2 -> PID Attitude/1(Entrée)
  Calcul J^-1/1(J^-1) -> Product1/1
  Reshape3/1 -> Product2/2
  Product1/1 -> Reshape3/1
  Product2/1 -> Reshape4/1
  Reshape4/1 -> Mux/2
  Reshape5/1 -> Mux/1
  PID Attitude/1(Sortie) -> Reshape2/1
  PID Position/1(Sortie) -> Reshape/1
  Constant2/1 -> Product2/1
  Gain/1 -> Euler Angles to  Direction Cosine Matrix/1
  Euler Angles to  Direction Cosine Matrix/1 -> Product/1
  Reshape/1 -> Product/2

== system drone/Mecanique/Mise en forme1 ==
  Entree : Inport  Port=1  LatchInput=off
  Demux2 : Demux  Outputs=2
  Mux1 : Mux  Inputs=2
  Reshape1 : simulink/Math Operations/Reshape  OutputDimensionality=1-D array  OutputDimensions=[1,1]
  Sortie : Outport
  wires:
  Entree/1 -> Demux2/1
  Mux1/1 -> Reshape1/1
  Demux2/2 -> Mux1/1
  Demux2/1 -> Mux1/2
  Reshape1/1 -> Sortie/1

== system drone/Mecanique/Mise en forme2 ==
  Entree : Inport  Port=1  LatchInput=off
  Demux2 : Demux  Outputs=2
  Mux1 : Mux  Inputs=2
  Reshape1 : simulink/Math Operations/Reshape  OutputDimensionality=1-D array  OutputDimensions=[1,1]
  Sortie : Outport
  wires:
  Reshape1/1 -> Sortie/1
  Demux2/1 -> Mux1/2
  Demux2/2 -> Mux1/1
  Mux1/1 -> Reshape1/1
  Entree/1 -> Demux2/1

== system drone/Mecanique/Mise en forme3 ==
  Entree : Inport  Port=1  LatchInput=off
  Demux2 : Demux  Outputs=2
  Mux1 : Mux  Inputs=2
  Reshape1 : simulink/Math Operations/Reshape  OutputDimensionality=1-D array  OutputDimensions=[1,1]
  Sortie : Outport
  wires:
  Entree/1 -> Demux2/1
  Mux1/1 -> Reshape1/1
  Demux2/2 -> Mux1/1
  Demux2/1 -> Mux1/2
  Reshape1/1 -> Sortie/1

== system drone/Mecanique/Mise en forme4 ==
  Entree : Inport  Port=1  LatchInput=off
  Demux2 : Demux  Outputs=2
  Mux1 : Mux  Inputs=2
  Reshape1 : simulink/Math Operations/Reshape  OutputDimensionality=1-D array  OutputDimensions=[1,1]
  Sortie : Outport
  wires:
  Reshape1/1 -> Sortie/1
  Demux2/1 -> Mux1/2
  Demux2/2 -> Mux1/1
  Mux1/1 -> Reshape1/1
  Entree/1 -> Demux2/1

== system drone/Utilisateur/Generateur F ==
  Demux : Demux  Tag=STV Demux  Outputs=6
  FromWs : FromWorkspace  Tag=STV FromWs  VariableName=tuvar  SampleTime=0  SigBuilderData=DataTag1  VnvData=DataTag2
      SigBuilderData=|
      | channels(1).label = 'X'
      | channels(1).allXData = {[0 1 1 2 2 15], [0 15], [0 8 8 11.5 11.5 15], [0 0.01 0.02 0.03 0.04 0.05 0.06 0.07 0.08 0.09 0.1 0.11 ... (1516 elements, 1x1516)]}
      | channels(1).allYData = {[0 0 1 1 0 0], [0 0], [0 0 1 1 0 0], [0 0.0627905195293 0.125333233564 0.187381314586 0.248689887165 0.309016994375 0.368124552685 0.425779291565 0.481753674102 0.535826794979 0.587785252292 0.637423989749 ... (1516 elements, 1x1516)]}
      | channels(2).label = 'Y'
      | channels(2).allXData = {[0 3 3 4 4 15], [0 15], [0 5 10 15], [0 0.01 0.02 0.03 0.04 0.05 0.06 0.07 0.08 0.09 0.1 0.11 ... (1516 elements, 1x1516)]}
      | channels(2).allYData = {[0 0 1 1 0 0], [0 0], [0 0 0 0], [0 0.0627905195293 0.125333233564 0.187381314586 0.248689887165 0.309016994375 0.368124552685 0.425779291565 0.481753674102 0.535826794979 0.587785252292 0.637423989749 ... (1516 elements, 1x1516)]}
      | channels(3).label = 'Z'
      | channels(3).allXData = {[0 5 5 6 6 15], [0 15], [0 5 10 15], [0 0.01 0.02 0.03 0.04 0.05 0.06 0.07 0.08 0.09 0.1 0.11 ... (1516 elements, 1x1516)]}
      | channels(3).allYData = {[0 0 1 1 0 0], [0 0], [0 0 0 0], [0 0.0627905195293 0.125333233564 0.187381314586 0.248689887165 0.309016994375 0.368124552685 0.425779291565 0.481753674102 0.535826794979 0.587785252292 0.637423989749 ... (1516 elements, 1x1516)]}
      | channels(4).label = 'Phi'
      | channels(4).allXData = {[0 7 7 8 8 15], [0 15], [0 3.5 10 15], [0 0.01 0.02 0.03 0.04 0.05 0.06 0.07 0.08 0.09 0.1 0.11 ... (1516 elements, 1x1516)]}
      | channels(4).allYData = {[0 0 1 1 0 0], [0 0], [0 0 0 0], [0 0.0627905195293 0.125333233564 0.187381314586 0.248689887165 0.309016994375 0.368124552685 0.425779291565 0.481753674102 0.535826794979 0.587785252292 0.637423989749 ... (1516 elements, 1x1516)]}
      | channels(5).label = 'Theta'
      | channels(5).allXData = {[0 9 9 10 10 15], [0 15], [0 5 10 15], [0 0.01 0.02 0.03 0.04 0.05 0.06 0.07 0.08 0.09 0.1 0.11 ... (1516 elements, 1x1516)]}
      | channels(5).allYData = {[0 0 1 1 0 0], [0 0], [0 0 0 0], [0 0.0627905195293 0.125333233564 0.187381314586 0.248689887165 0.309016994375 0.368124552685 0.425779291565 0.481753674102 0.535826794979 0.587785252292 0.637423989749 ... (1516 elements, 1x1516)]}
      | channels(6).label = 'Psi'
      | channels(6).allXData = {[0 11 11 12 12 15], [0 15], [0 1.5 1.5 5 5 15], [0 0.01 0.02 0.03 0.04 0.05 0.06 0.07 0.08 0.09 0.1 0.11 ... (1516 elements, 1x1516)]}
      | channels(6).allYData = {[0 0 1 1 0 0], [0 0], [0 0 1 1 0 0], [0 0.0627905195293 0.125333233564 0.187381314586 0.248689887165 0.309016994375 0.368124552685 0.425779291565 0.481753674102 0.535826794979 0.587785252292 0.637423989749 ... (1516 elements, 1x1516)]}
      | dataSet(1).timeRange = [0 15]
      | dataSet(1).name = 'Test General Validation'
      | dataSet(2).timeRange = [0 15]
      | dataSet(2).name = 'Neutre'
      | dataSet(3).timeRange = [0 15]
      | dataSet(3).name = 'Axe Principal'
      | dataSet(4).timeRange = [0 15]
      | dataSet(4).name = 'Test Harmonique'
  X : Outport  Tag=STV Outport
  Y : Outport  Tag=STV Outport  Port=2
  Z : Outport  Tag=STV Outport  Port=3
  Phi : Outport  Tag=STV Outport  Port=4
  Theta : Outport  Tag=STV Outport  Port=5
  Psi : Outport  Tag=STV Outport  Port=6
  wires:
  Demux/1 -> X/1
  FromWs/1 -> Demux/1
  Demux/2 -> Y/1
  Demux/3 -> Z/1
  Demux/4 -> Phi/1
  Demux/5 -> Theta/1
  Demux/6 -> Psi/1

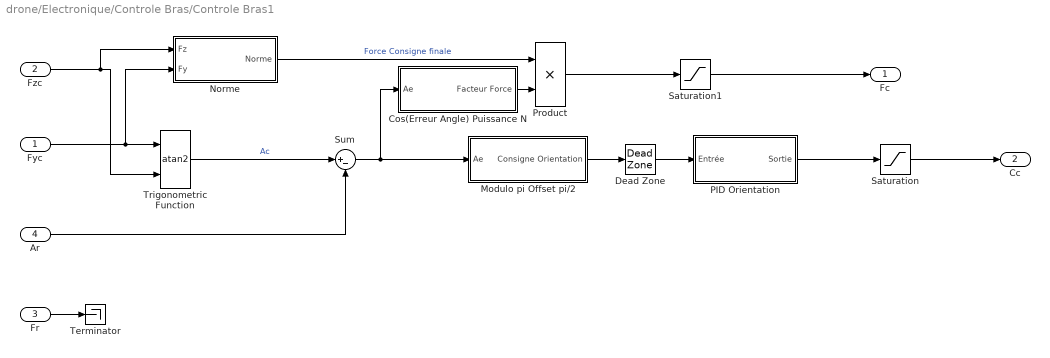
== system drone/Electronique/Controle Bras/Controle Bras1 ==
  Fyc : Inport  Port=1  LatchInput=off
  Fzc : Inport  Port=2  LatchInput=off
  Fr : Inport  Port=3  LatchInput=off
  Ar : Inport  Port=4  LatchInput=off
  Cos(Erreur Angle) Puissance N : Subsystem
  Dead Zone : DeadZone  LowerValue=-DZOrientation  UpperValue=DZOrientation  SaturateOnIntegerOverflow=on
  Modulo pi Offset pi/2 : Subsystem
  Norme : Subsystem
  PID Orientation : Subsystem
  Product : Product  RndMeth=Zero
  Saturation : Saturate
  Saturation1 : Saturate  UpperLimit=FrotorSat  LowerLimit=-FrotorSat
  Sum : Sum  Inputs=|+-
  Terminator : Terminator
  Trigonometric Function : Trigonometry  Operator=atan2  OutputSignalType=real
  Fc : Outport
  Cc : Outport  Port=2
  wires:
  Fzc/1 -> Trigonometric Function/2, Norme/1(Fz)
  Fyc/1 -> Trigonometric Function/1, Norme/2(Fy)
  Trigonometric Function/1 -> Sum/1  "Ac"
  Norme/1(Norme) -> Product/1  "Force Consigne finale"
  Ar/1 -> Sum/2
  Sum/1 -> Modulo pi Offset pi/2/1(Ae), Cos(Erreur Angle) Puissance N/1(Ae)
  Fr/1 -> Terminator/1
  Cos(Erreur Angle) Puissance N/1(Facteur Force) -> Product/2
  Product/1 -> Saturation1/1
  Modulo pi Offset pi/2/1(Consigne Orientation) -> Dead Zone/1
  Saturation/1 -> Cc/1
  PID Orientation/1(Sortie) -> Saturation/1
  Saturation1/1 -> Fc/1
  Dead Zone/1 -> PID Orientation/1(Entrée)

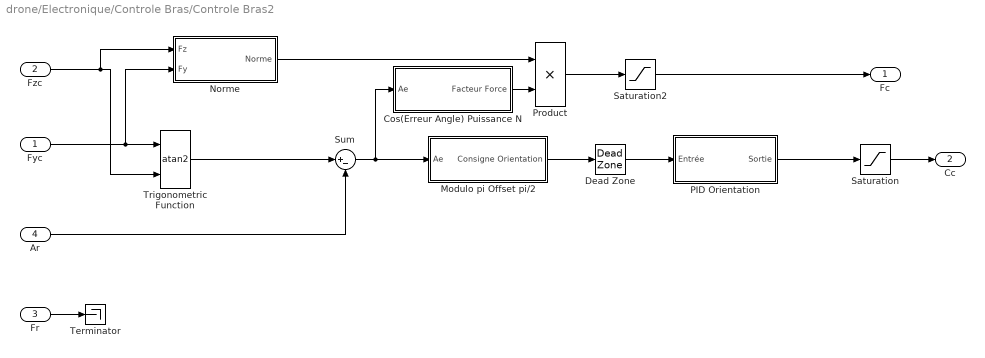
== system drone/Electronique/Controle Bras/Controle Bras2 ==
  Fyc : Inport  Port=1  LatchInput=off
  Fzc : Inport  Port=2  LatchInput=off
  Fr : Inport  Port=3  LatchInput=off
  Ar : Inport  Port=4  LatchInput=off
  Cos(Erreur Angle) Puissance N : Subsystem
  Dead Zone : DeadZone  LowerValue=-DZOrientation  UpperValue=DZOrientation  SaturateOnIntegerOverflow=on
  Modulo pi Offset pi/2 : Subsystem
  Norme : Subsystem
  PID Orientation : Subsystem
  Product : Product  RndMeth=Zero
  Saturation : Saturate
  Saturation2 : Saturate  UpperLimit=FrotorSat  LowerLimit=-FrotorSat
  Sum : Sum  Inputs=|+-
  Terminator : Terminator
  Trigonometric Function : Trigonometry  Operator=atan2  OutputSignalType=real
  Fc : Outport
  Cc : Outport  Port=2
  wires:
  Fzc/1 -> Trigonometric Function/2, Norme/1(Fz)
  Fyc/1 -> Trigonometric Function/1, Norme/2(Fy)
  Trigonometric Function/1 -> Sum/1
  Norme/1(Norme) -> Product/1
  Ar/1 -> Sum/2
  Sum/1 -> Modulo pi Offset pi/2/1(Ae), Cos(Erreur Angle) Puissance N/1(Ae)
  Fr/1 -> Terminator/1
  Product/1 -> Saturation2/1
  Modulo pi Offset pi/2/1(Consigne Orientation) -> Dead Zone/1
  Saturation/1 -> Cc/1
  Cos(Erreur Angle) Puissance N/1(Facteur Force) -> Product/2
  PID Orientation/1(Sortie) -> Saturation/1
  Saturation2/1 -> Fc/1
  Dead Zone/1 -> PID Orientation/1(Entrée)

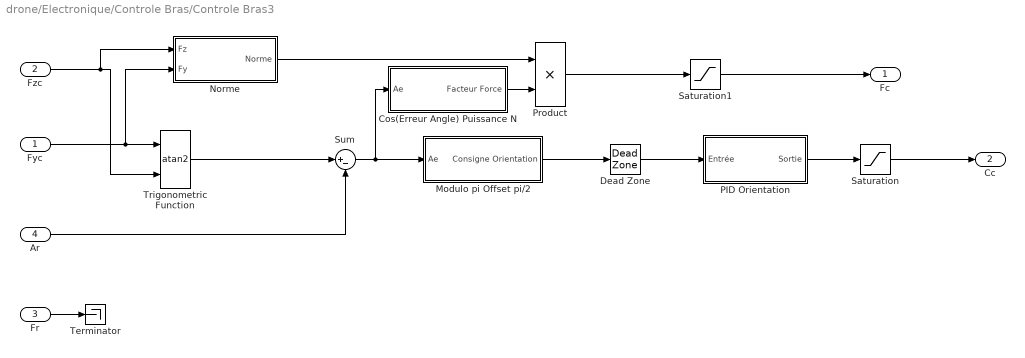
== system drone/Electronique/Controle Bras/Controle Bras3 ==
  Fyc : Inport  Port=1  LatchInput=off
  Fzc : Inport  Port=2  LatchInput=off
  Fr : Inport  Port=3  LatchInput=off
  Ar : Inport  Port=4  LatchInput=off
  Cos(Erreur Angle) Puissance N : Subsystem
  Dead Zone : DeadZone  LowerValue=-DZOrientation  UpperValue=DZOrientation  SaturateOnIntegerOverflow=on
  Modulo pi Offset pi/2 : Subsystem
  Norme : Subsystem
  PID Orientation : Subsystem
  Product : Product  RndMeth=Zero
  Saturation : Saturate
  Saturation1 : Saturate  UpperLimit=FrotorSat  LowerLimit=-FrotorSat
  Sum : Sum  Inputs=|+-
  Terminator : Terminator
  Trigonometric Function : Trigonometry  Operator=atan2  OutputSignalType=real
  Fc : Outport
  Cc : Outport  Port=2
  wires:
  Fzc/1 -> Trigonometric Function/2, Norme/1(Fz)
  Fyc/1 -> Trigonometric Function/1, Norme/2(Fy)
  Trigonometric Function/1 -> Sum/1
  Norme/1(Norme) -> Product/1
  Ar/1 -> Sum/2
  Sum/1 -> Modulo pi Offset pi/2/1(Ae), Cos(Erreur Angle) Puissance N/1(Ae)
  PID Orientation/1(Sortie) -> Saturation/1
  Fr/1 -> Terminator/1
  Product/1 -> Saturation1/1
  Modulo pi Offset pi/2/1(Consigne Orientation) -> Dead Zone/1
  Saturation/1 -> Cc/1
  Cos(Erreur Angle) Puissance N/1(Facteur Force) -> Product/2
  Saturation1/1 -> Fc/1
  Dead Zone/1 -> PID Orientation/1(Entrée)

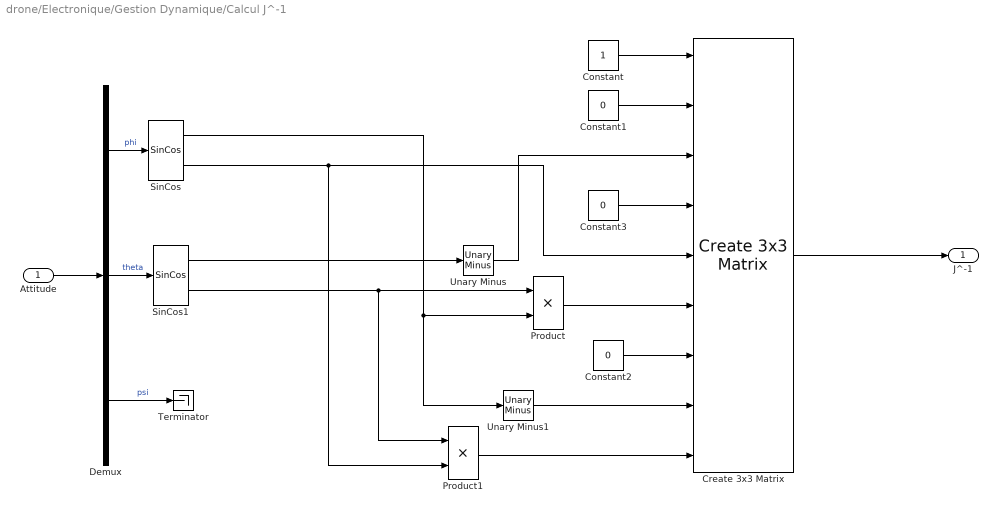
== system drone/Electronique/Gestion Dynamique/Calcul J^-1 ==
  Attitude : Inport  Port=1  LatchInput=off
  Constant : Constant
  Constant1 : Constant  Value=0
  Constant2 : Constant  Value=0
  Constant3 : Constant  Value=0
  Create 3x3 Matrix : aerolibutil/Create 3x3 Matrix
  Demux : Demux  Outputs=3
  Product : Product  RndMeth=Zero
  Product1 : Product  RndMeth=Zero
  SinCos : aerolibutil/SinCos
  SinCos1 : aerolibutil/SinCos
  Terminator : Terminator
  Unary Minus : simulink/Math Operations/Unary Minus  DoSatur=off
  Unary Minus1 : simulink/Math Operations/Unary Minus  DoSatur=off
  J^-1 : Outport
      settings: BusObject=perturbations
  wires:
  Attitude/1 -> Demux/1
  Create 3x3 Matrix/1 -> J^-1/1
  Demux/1 -> SinCos/1  "phi"
  Demux/2 -> SinCos1/1  "theta"
  Constant/1 -> Create 3x3 Matrix/1
  Constant1/1 -> Create 3x3 Matrix/2
  SinCos1/1 -> Unary Minus/1
  Demux/3 -> Terminator/1  "psi"
  Constant3/1 -> Create 3x3 Matrix/4
  Constant2/1 -> Create 3x3 Matrix/7
  SinCos/2 -> Create 3x3 Matrix/5, Product1/2
  SinCos/1 -> Product/2, Unary Minus1/1
  SinCos1/2 -> Product/1, Product1/1
  Product/1 -> Create 3x3 Matrix/6
  Product1/1 -> Create 3x3 Matrix/9
  Unary Minus/1 -> Create 3x3 Matrix/3
  Unary Minus1/1 -> Create 3x3 Matrix/8

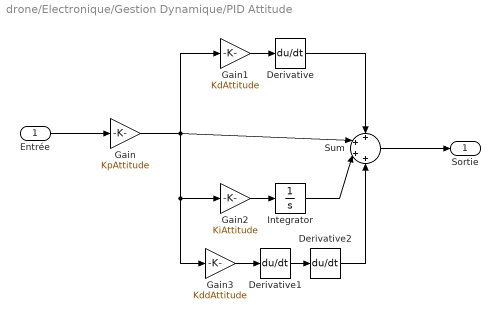
== system drone/Electronique/Gestion Dynamique/PID Attitude ==
  Entrée : Inport  Port=1  LatchInput=off
  Derivative : Derivative
  Derivative1 : Derivative
  Derivative2 : Derivative
  Gain : Gain  Gain=KpAttitude
  Gain1 : Gain  Gain=KdAttitude
  Gain2 : Gain  Gain=KiAttitude
  Gain3 : Gain  Gain=KddAttitude
  Integrator : Integrator
  Sum : Sum  Inputs=++++
  Sortie : Outport
      settings: BusObject=perturbations
  wires:
  Entrée/1 -> Gain/1
  Gain/1 -> Sum/2, Gain1/1, Gain2/1, Gain3/1
  Derivative/1 -> Sum/1
  Integrator/1 -> Sum/3
  Gain2/1 -> Integrator/1
  Gain1/1 -> Derivative/1
  Sum/1 -> Sortie/1
  Gain3/1 -> Derivative1/1
  Derivative1/1 -> Derivative2/1
  Derivative2/1 -> Sum/4

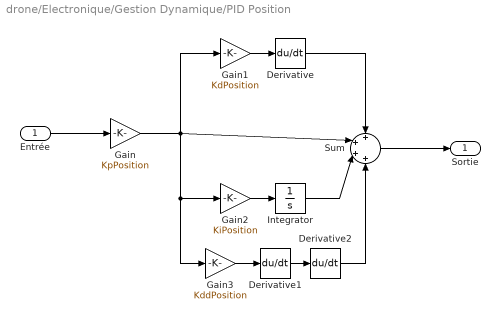
== system drone/Electronique/Gestion Dynamique/PID Position ==
  Entrée : Inport  Port=1  LatchInput=off
  Derivative : Derivative
  Derivative1 : Derivative
  Derivative2 : Derivative
  Gain : Gain  Gain=KpPosition
  Gain1 : Gain  Gain=KdPosition
  Gain2 : Gain  Gain=KiPosition
  Gain3 : Gain  Gain=KddPosition
  Integrator : Integrator
  Sum : Sum  Inputs=++++
  Sortie : Outport
      settings: BusObject=perturbations
  wires:
  Entrée/1 -> Gain/1
  Gain/1 -> Sum/2, Gain1/1, Gain2/1, Gain3/1
  Derivative/1 -> Sum/1
  Integrator/1 -> Sum/3
  Gain2/1 -> Integrator/1
  Gain1/1 -> Derivative/1
  Sum/1 -> Sortie/1
  Gain3/1 -> Derivative1/1
  Derivative1/1 -> Derivative2/1
  Derivative2/1 -> Sum/4

== system drone/Electronique/Controle Bras/Controle Bras1/Cos(Erreur Angle) Puissance N ==
  Ae : Inport  Port=1  LatchInput=off
  Constant : Constant  Value=(ExposantFacteurAngulaire*2)+1
  Cos(Erreur  Angle) : Trigonometry  Operator=cos
  Math Function : Math  Operator=pow  SaturateOnIntegerOverflow=on
  Facteur Force : Outport
  wires:
  Ae/1 -> Cos(Erreur  Angle)/1
  Cos(Erreur  Angle)/1 -> Math Function/1
  Constant/1 -> Math Function/2
  Math Function/1 -> Facteur Force/1

== system drone/Electronique/Controle Bras/Controle Bras1/Modulo pi Offset pi/2 ==
  Ae : Inport  Port=1  LatchInput=off
  Constant : Constant  Value=pi
  Constant1 : Constant  Value=pi/2
  Constant2 : Constant  Value=pi/2
  Math Function : Math  Operator=mod  SaturateOnIntegerOverflow=on
  Sum : Sum  Inputs=|++
  Sum1 : Sum  Inputs=|+-
  Consigne Orientation : Outport
  wires:
  Constant/1 -> Math Function/2
  Sum/1 -> Math Function/1
  Constant1/1 -> Sum/2
  Ae/1 -> Sum/1
  Constant2/1 -> Sum1/2
  Math Function/1 -> Sum1/1
  Sum1/1 -> Consigne Orientation/1

== system drone/Electronique/Controle Bras/Controle Bras1/Norme ==
  Fz : Inport  Port=1  LatchInput=off
  Fy : Inport  Port=2  LatchInput=off
  Add : Sum  OutScaling=2^-10
  Math Function : Math  Operator=square  SaturateOnIntegerOverflow=on
  Math Function1 : Math  Operator=square  SaturateOnIntegerOverflow=on
  Math Function2 : Math  Operator=sqrt  SaturateOnIntegerOverflow=on
  Norme : Outport
  wires:
  Add/1 -> Math Function2/1
  Math Function1/1 -> Add/1
  Math Function/1 -> Add/2
  Fz/1 -> Math Function1/1
  Fy/1 -> Math Function/1
  Math Function2/1 -> Norme/1

== system drone/Electronique/Controle Bras/Controle Bras1/PID Orientation ==
  Entrée : Inport  Port=1  LatchInput=off
  Derivative : Derivative
  Gain : Gain  Gain=KpOrientation
  Gain1 : Gain  Gain=KdOrientation
  Gain2 : Gain  Gain=KiOrientation
  Integrator : Integrator
  Sum : Sum  Inputs=+++
  Sortie : Outport
      settings: BusObject=perturbations
  wires:
  Entrée/1 -> Gain/1
  Gain/1 -> Sum/2, Gain1/1, Gain2/1
  Derivative/1 -> Sum/1
  Integrator/1 -> Sum/3
  Gain2/1 -> Integrator/1
  Gain1/1 -> Derivative/1
  Sum/1 -> Sortie/1

== system drone/Electronique/Controle Bras/Controle Bras2/Cos(Erreur Angle) Puissance N ==
  Ae : Inport  Port=1  LatchInput=off
  Constant : Constant  Value=(ExposantFacteurAngulaire*2)+1
  Cos(Erreur  Angle) : Trigonometry  Operator=cos
  Math Function : Math  Operator=pow  SaturateOnIntegerOverflow=on
  Facteur Force : Outport
  wires:
  Ae/1 -> Cos(Erreur  Angle)/1
  Cos(Erreur  Angle)/1 -> Math Function/1
  Constant/1 -> Math Function/2
  Math Function/1 -> Facteur Force/1

== system drone/Electronique/Controle Bras/Controle Bras2/Modulo pi Offset pi/2 ==
  Ae : Inport  Port=1  LatchInput=off
  Constant : Constant  Value=pi
  Constant1 : Constant  Value=pi/2
  Constant2 : Constant  Value=pi/2
  Math Function : Math  Operator=mod  SaturateOnIntegerOverflow=on
  Sum : Sum  Inputs=|++
  Sum1 : Sum  Inputs=|+-
  Consigne Orientation : Outport
  wires:
  Constant/1 -> Math Function/2
  Sum/1 -> Math Function/1
  Constant1/1 -> Sum/2
  Ae/1 -> Sum/1
  Constant2/1 -> Sum1/2
  Math Function/1 -> Sum1/1
  Sum1/1 -> Consigne Orientation/1

== system drone/Electronique/Controle Bras/Controle Bras2/Norme ==
  Fz : Inport  Port=1  LatchInput=off
  Fy : Inport  Port=2  LatchInput=off
  Add : Sum  OutScaling=2^-10
  Math Function : Math  Operator=square  SaturateOnIntegerOverflow=on
  Math Function1 : Math  Operator=square  SaturateOnIntegerOverflow=on
  Math Function2 : Math  Operator=sqrt  SaturateOnIntegerOverflow=on
  Norme : Outport
  wires:
  Add/1 -> Math Function2/1
  Math Function1/1 -> Add/1
  Math Function/1 -> Add/2
  Fz/1 -> Math Function1/1
  Fy/1 -> Math Function/1
  Math Function2/1 -> Norme/1

== system drone/Electronique/Controle Bras/Controle Bras2/PID Orientation ==
  Entrée : Inport  Port=1  LatchInput=off
  Derivative : Derivative
  Gain : Gain  Gain=KpOrientation
  Gain1 : Gain  Gain=KdOrientation
  Gain2 : Gain  Gain=KiOrientation
  Integrator : Integrator
  Sum : Sum  Inputs=+++
  Sortie : Outport
      settings: BusObject=perturbations
  wires:
  Entrée/1 -> Gain/1
  Gain/1 -> Sum/2, Gain1/1, Gain2/1
  Derivative/1 -> Sum/1
  Integrator/1 -> Sum/3
  Gain2/1 -> Integrator/1
  Gain1/1 -> Derivative/1
  Sum/1 -> Sortie/1

== system drone/Electronique/Controle Bras/Controle Bras3/Cos(Erreur Angle) Puissance N ==
  Ae : Inport  Port=1  LatchInput=off
  Constant : Constant  Value=(ExposantFacteurAngulaire*2)+1
  Cos(Erreur  Angle) : Trigonometry  Operator=cos
  Math Function : Math  Operator=pow  SaturateOnIntegerOverflow=on
  Facteur Force : Outport
  wires:
  Ae/1 -> Cos(Erreur  Angle)/1
  Cos(Erreur  Angle)/1 -> Math Function/1
  Constant/1 -> Math Function/2
  Math Function/1 -> Facteur Force/1

== system drone/Electronique/Controle Bras/Controle Bras3/Modulo pi Offset pi/2 ==
  Ae : Inport  Port=1  LatchInput=off
  Constant : Constant  Value=pi
  Constant1 : Constant  Value=pi/2
  Constant2 : Constant  Value=pi/2
  Math Function : Math  Operator=mod  SaturateOnIntegerOverflow=on
  Sum : Sum  Inputs=|++
  Sum1 : Sum  Inputs=|+-
  Consigne Orientation : Outport
  wires:
  Constant/1 -> Math Function/2
  Sum/1 -> Math Function/1
  Constant1/1 -> Sum/2
  Ae/1 -> Sum/1
  Constant2/1 -> Sum1/2
  Math Function/1 -> Sum1/1
  Sum1/1 -> Consigne Orientation/1

== system drone/Electronique/Controle Bras/Controle Bras3/Norme ==
  Fz : Inport  Port=1  LatchInput=off
  Fy : Inport  Port=2  LatchInput=off
  Add : Sum  OutScaling=2^-10
  Math Function : Math  Operator=square  SaturateOnIntegerOverflow=on
  Math Function1 : Math  Operator=square  SaturateOnIntegerOverflow=on
  Math Function2 : Math  Operator=sqrt  SaturateOnIntegerOverflow=on
  Norme : Outport
  wires:
  Add/1 -> Math Function2/1
  Math Function1/1 -> Add/1
  Math Function/1 -> Add/2
  Fz/1 -> Math Function1/1
  Fy/1 -> Math Function/1
  Math Function2/1 -> Norme/1

== system drone/Electronique/Controle Bras/Controle Bras3/PID Orientation ==
  Entrée : Inport  Port=1  LatchInput=off
  Derivative : Derivative
  Gain : Gain  Gain=KpOrientation
  Gain1 : Gain  Gain=KdOrientation
  Gain2 : Gain  Gain=KiOrientation
  Integrator : Integrator
  Sum : Sum  Inputs=+++
  Sortie : Outport
      settings: BusObject=perturbations
  wires:
  Entrée/1 -> Gain/1
  Gain/1 -> Sum/2, Gain1/1, Gain2/1
  Derivative/1 -> Sum/1
  Integrator/1 -> Sum/3
  Gain2/1 -> Integrator/1
  Gain1/1 -> Derivative/1
  Sum/1 -> Sortie/1
